simulink model "system4report"  (R2015b)
settings: Solver=VariableStepAuto  StartTime=0.0  StopTime=3  MaxStep=0.01  RelTol=1e-3
settings Model: Creator=kazuhiro  LastModifiedBy=kazuhiro

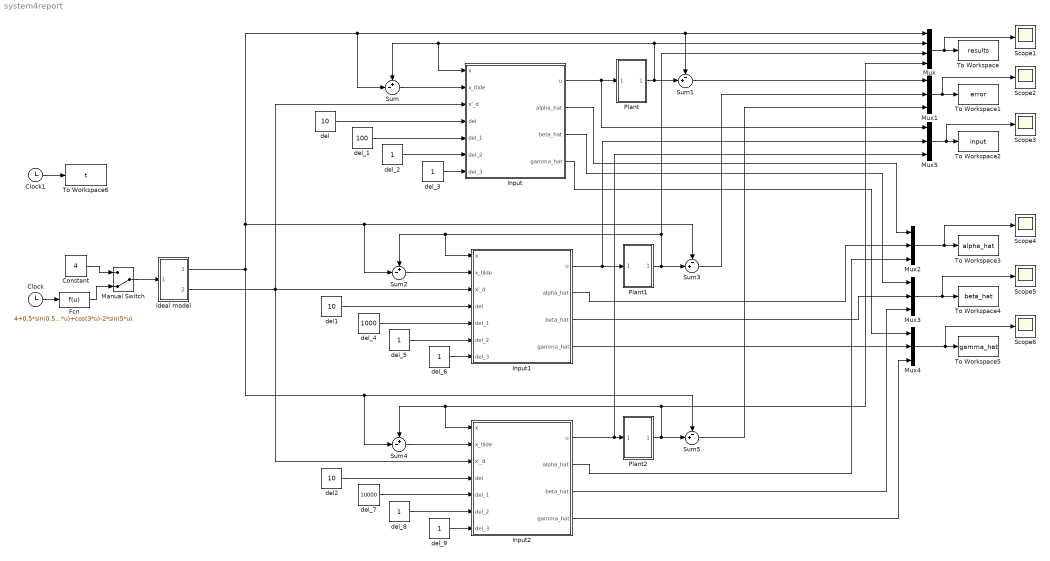
== system system4report ==
  Clock : Clock
  Clock1 : Clock
  Constant : Constant  Value=4
  Fcn : Fcn  Expr=4+0.5*sin(0.5*u)+cos(3*u)-2*sin(5*u)
  Ideal model : Subsystem
  Input : Subsystem
  Input1 : Subsystem
  Input2 : Subsystem
  Manual Switch : ManualSwitch  CurrentSetting=0
  Mux : Mux
  Mux{1..5} (5 alike) : Mux  Inputs=3
  Plant : Subsystem
  Plant1 : Subsystem
  Plant2 : Subsystem
  Scope{1..6} (6 alike) : Scope
  Sum : Sum  Inputs=+-|
  Sum1 : Sum  Inputs=-+|
  Sum2 : Sum  Inputs=+-|
  Sum3 : Sum  Inputs=-+|
  Sum4 : Sum  Inputs=+-|
  Sum5 : Sum  Inputs=-+|
  To Workspace : ToWorkspace  VariableName=results  SampleTime=-1
  To Workspace1 : ToWorkspace  VariableName=error  SampleTime=-1
  To Workspace2 : ToWorkspace  VariableName=input  SampleTime=-1
  To Workspace3 : ToWorkspace  VariableName=alpha_hat  SampleTime=-1
  To Workspace4 : ToWorkspace  VariableName=beta_hat  SampleTime=-1
  To Workspace5 : ToWorkspace  VariableName=gamma_hat  SampleTime=-1
  To Workspace6 : ToWorkspace  VariableName=t  SampleTime=-1
  del : Constant  Value=10
  del1 : Constant  Value=10
  del2 : Constant  Value=10
  del_1 : Constant  Value=100
  del_{2..3,5..6,8..9} (6 alike) : Constant
  del_4 : Constant  Value=1000
  del_7 : Constant  Value=10000
  wires:
  Input/1(u) -> Mux5/1, Plant/1(u(t))
  Manual Switch/1 -> Ideal model/1(r_d)
  Constant/1 -> Manual Switch/1
  Clock/1 -> Fcn/1
  Fcn/1 -> Manual Switch/2
  del/1 -> Input/4("del ")
  del_2/1 -> Input/6(del_2)
  del_3/1 -> Input/7(del_3)
  Plant/1(x(t)) -> Mux/2, Sum/1, Input/1(x), Sum1/2
  del_1/1 -> Input/5(del_1)
  Sum/1 -> Input/2(x_tilde)
  Mux/1 -> Scope1/1, To Workspace/1
  Sum1/1 -> Mux1/1
  Input/2(alpha_hat) -> Mux2/1
  Input/3(beta_hat) -> Mux3/1
  Input/4(gamma_hat) -> Mux4/1
  Input1/1(u) -> Plant1/1(u(t)), Mux5/2
  del1/1 -> Input1/4("del ")
  del_5/1 -> Input1/6(del_2)
  del_6/1 -> Input1/7(del_3)
  Plant1/1(x(t)) -> Sum3/2, Mux/3, Sum2/1, Input1/1(x)
  del_4/1 -> Input1/5(del_1)
  Sum2/1 -> Input1/2(x_tilde)
  Sum3/1 -> Mux1/2
  Input1/2(alpha_hat) -> Mux2/2
  Input1/3(beta_hat) -> Mux3/2
  Input1/4(gamma_hat) -> Mux4/2
  Mux2/1 -> Scope4/1, To Workspace3/1
  Mux3/1 -> Scope5/1, To Workspace4/1
  Mux4/1 -> Scope6/1, To Workspace5/1
  Mux1/1 -> Scope2/1, To Workspace1/1
  Mux5/1 -> Scope3/1, To Workspace2/1
  Input2/1(u) -> Mux5/3, Plant2/1(u(t))
  Ideal model/2(x'_d) -> Input2/3(x'_d), Input/3(x'_d), Input1/3(x'_d)
  del2/1 -> Input2/4("del ")
  del_8/1 -> Input2/6(del_2)
  del_9/1 -> Input2/7(del_3)
  Plant2/1(x(t)) -> Mux/4, Input2/1(x), Sum4/1, Sum5/2
  Ideal model/1(x_d) -> Sum4/2, Sum5/1, Sum/2, Sum1/1, Mux/1, Sum3/1, Sum2/2
  del_7/1 -> Input2/5(del_1)
  Sum4/1 -> Input2/2(x_tilde)
  Sum5/1 -> Mux1/3
  Input2/2(alpha_hat) -> Mux2/3
  Input2/3(beta_hat) -> Mux3/3
  Input2/4(gamma_hat) -> Mux4/3
  Clock1/1 -> To Workspace6/1

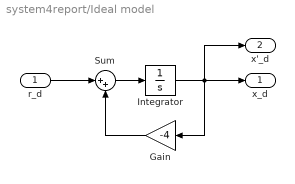
== system system4report/Ideal model ==
  r_d : Inport
  Gain : Gain  Gain=-4
  Integrator : Integrator
  Sum : Sum  Inputs=|++
  x_d : Outport
  x'_d : Outport  Port=2
  wires:
  Gain/1 -> Sum/2
  r_d/1 -> Sum/1
  Integrator/1 -> x_d/1, Gain/1, x'_d/1
  Sum/1 -> Integrator/1

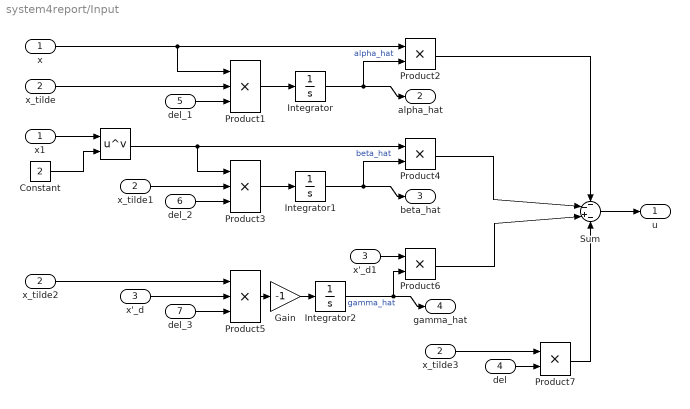
== system system4report/Input ==
  x : Inport
  x_tilde : Inport  Port=2
  x'_d : Inport  Port=3
  "del " : Inport  Port=4
  del_1 : Inport  Port=5
  del_2 : Inport  Port=6
  del_3 : Inport  Port=7
  " " : Math  Operator=pow  SaturateOnIntegerOverflow=on
  Constant : Constant  Value=2
  Gain : Gain  Gain=-1
  Integrator : Integrator
  Integrator1 : Integrator
  Integrator2 : Integrator
  Product1 : Product  Inputs=3
  Product{2,4,6..7} (4 alike) : Product
  Product3 : Product  Inputs=3
  Product5 : Product  Inputs=3
  Sum : Sum  Inputs=--+-
  x'_d1 : InportShadow  Port=3
  x1 : InportShadow
  x_tilde1 : InportShadow  Port=2
  x_tilde2 : InportShadow  Port=2
  x_tilde3 : InportShadow  Port=2
  u : Outport
  alpha_hat : Outport  Port=2
  beta_hat : Outport  Port=3
  gamma_hat : Outport  Port=4
  wires:
  Product2/1 -> Sum/1
  x_tilde/1 -> Product1/2
  x/1 -> Product2/1, Product1/1
  Integrator/1 -> alpha_hat/1, Product2/2  "alpha_hat"
  Product1/1 -> Integrator/1
  del_1/1 -> Product1/3
  Product4/1 -> Sum/2
  x_tilde1/1 -> Product3/2
  " "/1 -> Product3/1, Product4/1
  Integrator1/1 -> Product4/2, beta_hat/1  "beta_hat"
  Product3/1 -> Integrator1/1
  del_2/1 -> Product3/3
  x1/1 -> " "/1
  Constant/1 -> " "/2
  Product6/1 -> Sum/3
  x'_d/1 -> Product5/2
  Integrator2/1 -> gamma_hat/1, Product6/2  "gamma_hat"
  del_3/1 -> Product5/3
  Product5/1 -> Gain/1
  Gain/1 -> Integrator2/1
  x'_d1/1 -> Product6/1
  "del "/1 -> Product7/2
  x_tilde2/1 -> Product5/1
  x_tilde3/1 -> Product7/1
  Product7/1 -> Sum/4
  Sum/1 -> u/1

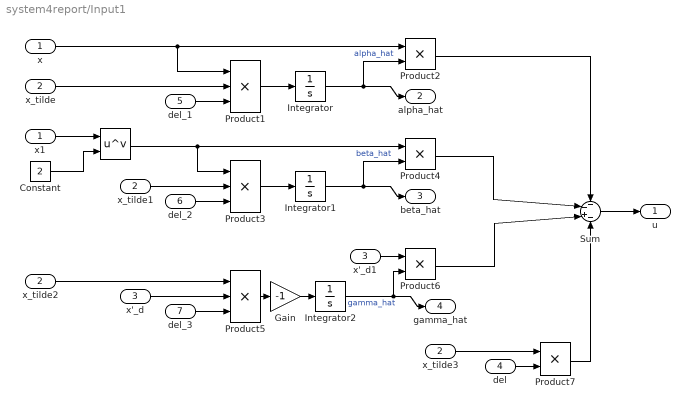
== system system4report/Input1 ==
  x : Inport
  x_tilde : Inport  Port=2
  x'_d : Inport  Port=3
  "del " : Inport  Port=4
  del_1 : Inport  Port=5
  del_2 : Inport  Port=6
  del_3 : Inport  Port=7
  " " : Math  Operator=pow  SaturateOnIntegerOverflow=on
  Constant : Constant  Value=2
  Gain : Gain  Gain=-1
  Integrator : Integrator
  Integrator1 : Integrator
  Integrator2 : Integrator
  Product1 : Product  Inputs=3
  Product{2,4,6..7} (4 alike) : Product
  Product3 : Product  Inputs=3
  Product5 : Product  Inputs=3
  Sum : Sum  Inputs=--+-
  x'_d1 : InportShadow  Port=3
  x1 : InportShadow
  x_tilde1 : InportShadow  Port=2
  x_tilde2 : InportShadow  Port=2
  x_tilde3 : InportShadow  Port=2
  u : Outport
  alpha_hat : Outport  Port=2
  beta_hat : Outport  Port=3
  gamma_hat : Outport  Port=4
  wires:
  Sum/1 -> u/1
  Product7/1 -> Sum/4
  x_tilde3/1 -> Product7/1
  x_tilde2/1 -> Product5/1
  "del "/1 -> Product7/2
  x'_d1/1 -> Product6/1
  Gain/1 -> Integrator2/1
  Product5/1 -> Gain/1
  del_3/1 -> Product5/3
  Integrator2/1 -> Product6/2, gamma_hat/1  "gamma_hat"
  x'_d/1 -> Product5/2
  Product6/1 -> Sum/3
  Constant/1 -> " "/2
  x1/1 -> " "/1
  del_2/1 -> Product3/3
  Product3/1 -> Integrator1/1
  Integrator1/1 -> beta_hat/1, Product4/2  "beta_hat"
  " "/1 -> Product4/1, Product3/1
  x_tilde1/1 -> Product3/2
  Product4/1 -> Sum/2
  del_1/1 -> Product1/3
  Product1/1 -> Integrator/1
  Integrator/1 -> Product2/2, alpha_hat/1  "alpha_hat"
  x/1 -> Product1/1, Product2/1
  x_tilde/1 -> Product1/2
  Product2/1 -> Sum/1

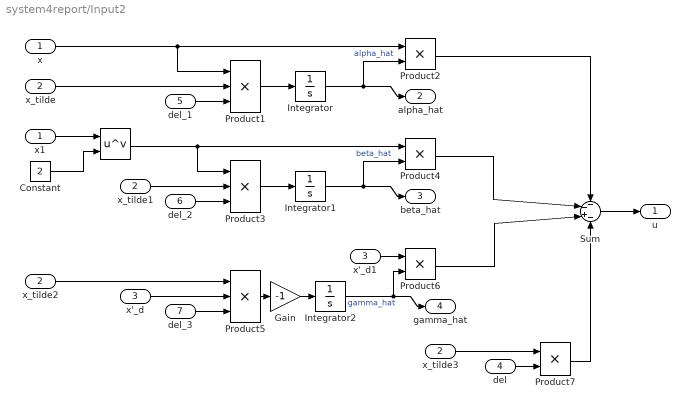
== system system4report/Input2 ==
  x : Inport
  x_tilde : Inport  Port=2
  x'_d : Inport  Port=3
  "del " : Inport  Port=4
  del_1 : Inport  Port=5
  del_2 : Inport  Port=6
  del_3 : Inport  Port=7
  " " : Math  Operator=pow  SaturateOnIntegerOverflow=on
  Constant : Constant  Value=2
  Gain : Gain  Gain=-1
  Integrator : Integrator
  Integrator1 : Integrator
  Integrator2 : Integrator
  Product1 : Product  Inputs=3
  Product{2,4,6..7} (4 alike) : Product
  Product3 : Product  Inputs=3
  Product5 : Product  Inputs=3
  Sum : Sum  Inputs=--+-
  x'_d1 : InportShadow  Port=3
  x1 : InportShadow
  x_tilde1 : InportShadow  Port=2
  x_tilde2 : InportShadow  Port=2
  x_tilde3 : InportShadow  Port=2
  u : Outport
  alpha_hat : Outport  Port=2
  beta_hat : Outport  Port=3
  gamma_hat : Outport  Port=4
  wires:
  Product2/1 -> Sum/1
  x_tilde/1 -> Product1/2
  x/1 -> Product2/1, Product1/1
  Integrator/1 -> alpha_hat/1, Product2/2  "alpha_hat"
  Product1/1 -> Integrator/1
  del_1/1 -> Product1/3
  Product4/1 -> Sum/2
  x_tilde1/1 -> Product3/2
  " "/1 -> Product3/1, Product4/1
  Integrator1/1 -> Product4/2, beta_hat/1  "beta_hat"
  Product3/1 -> Integrator1/1
  del_2/1 -> Product3/3
  x1/1 -> " "/1
  Constant/1 -> " "/2
  Product6/1 -> Sum/3
  x'_d/1 -> Product5/2
  Integrator2/1 -> gamma_hat/1, Product6/2  "gamma_hat"
  del_3/1 -> Product5/3
  Product5/1 -> Gain/1
  Gain/1 -> Integrator2/1
  x'_d1/1 -> Product6/1
  "del "/1 -> Product7/2
  x_tilde2/1 -> Product5/1
  x_tilde3/1 -> Product7/1
  Product7/1 -> Sum/4
  Sum/1 -> u/1

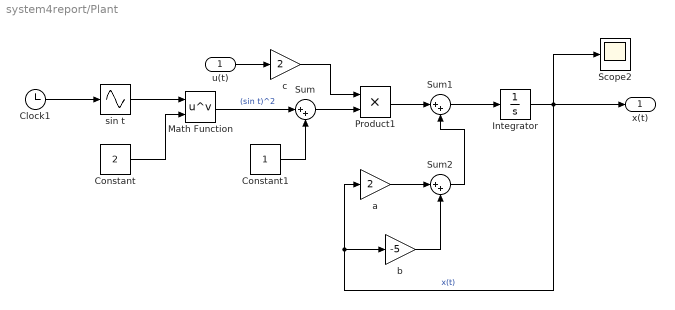
== system system4report/Plant ==
  u(t) : Inport
  Clock1 : Clock
  Constant : Constant  Value=2
  Constant1 : Constant
  Integrator : Integrator
  Math Function : Math  Operator=pow  SaturateOnIntegerOverflow=on
  Product1 : Product
  Scope2 : Scope
  Sum : Sum  Inputs=|++
  Sum1 : Sum  Inputs=|++
  Sum2 : Sum  Inputs=|++
  a : Gain  Gain=2
  b : Gain  Gain=-5
  "c " : Gain  Gain=2
  sin t : Sin  TimeSource=Use external signal  SampleTime=0
  x(t) : Outport
  wires:
  sin t/1 -> Math Function/1
  a/1 -> Sum2/1
  "c "/1 -> Product1/1
  Math Function/1 -> Sum/1  "(sin t)^2"
  b/1 -> Sum2/2
  u(t)/1 -> "c "/1
  Sum/1 -> Product1/2
  Sum1/1 -> Integrator/1
  Constant1/1 -> Sum/2
  Product1/1 -> Sum1/1
  Sum2/1 -> Sum1/2
  Integrator/1 -> a/1, b/1, x(t)/1, Scope2/1  "x(t)"
  Clock1/1 -> sin t/1
  Constant/1 -> Math Function/2

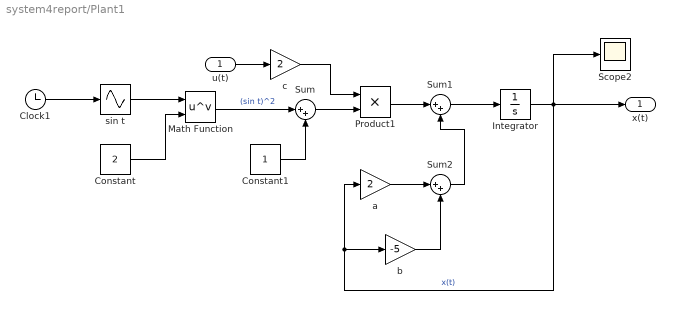
== system system4report/Plant1 ==
  u(t) : Inport
  Clock1 : Clock
  Constant : Constant  Value=2
  Constant1 : Constant
  Integrator : Integrator
  Math Function : Math  Operator=pow  SaturateOnIntegerOverflow=on
  Product1 : Product
  Scope2 : Scope
  Sum : Sum  Inputs=|++
  Sum1 : Sum  Inputs=|++
  Sum2 : Sum  Inputs=|++
  a : Gain  Gain=2
  b : Gain  Gain=-5
  "c " : Gain  Gain=2
  sin t : Sin  TimeSource=Use external signal  SampleTime=0
  x(t) : Outport
  wires:
  Constant/1 -> Math Function/2
  Clock1/1 -> sin t/1
  Integrator/1 -> Scope2/1, x(t)/1, b/1, a/1  "x(t)"
  Sum2/1 -> Sum1/2
  Product1/1 -> Sum1/1
  Constant1/1 -> Sum/2
  Sum1/1 -> Integrator/1
  Sum/1 -> Product1/2
  u(t)/1 -> "c "/1
  b/1 -> Sum2/2
  Math Function/1 -> Sum/1  "(sin t)^2"
  "c "/1 -> Product1/1
  a/1 -> Sum2/1
  sin t/1 -> Math Function/1

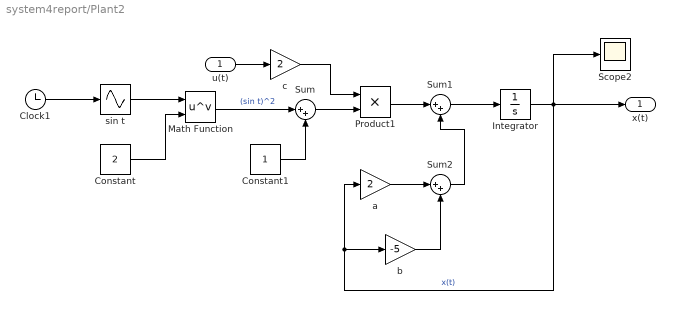
== system system4report/Plant2 ==
  u(t) : Inport
  Clock1 : Clock
  Constant : Constant  Value=2
  Constant1 : Constant
  Integrator : Integrator
  Math Function : Math  Operator=pow  SaturateOnIntegerOverflow=on
  Product1 : Product
  Scope2 : Scope
  Sum : Sum  Inputs=|++
  Sum1 : Sum  Inputs=|++
  Sum2 : Sum  Inputs=|++
  a : Gain  Gain=2
  b : Gain  Gain=-5
  "c " : Gain  Gain=2
  sin t : Sin  TimeSource=Use external signal  SampleTime=0
  x(t) : Outport
  wires:
  sin t/1 -> Math Function/1
  a/1 -> Sum2/1
  "c "/1 -> Product1/1
  Math Function/1 -> Sum/1  "(sin t)^2"
  b/1 -> Sum2/2
  u(t)/1 -> "c "/1
  Sum/1 -> Product1/2
  Sum1/1 -> Integrator/1
  Constant1/1 -> Sum/2
  Product1/1 -> Sum1/1
  Sum2/1 -> Sum1/2
  Integrator/1 -> a/1, b/1, x(t)/1, Scope2/1  "x(t)"
  Clock1/1 -> sin t/1
  Constant/1 -> Math Function/2
